simulink model "Ex3sim"  (R2024b)
settings: Solver=VariableStepAuto  StartTime=0.0  StopTime=10.0  RelTol=1e-3
values from neighbouring files (symbols this model uses):
  Ao = phi-L*H    [Ex2.m]    (also in Ex3.m; Extended_Estimator.m = Ae-L*Ce)
  Bo = [gamma L]    [Ex2.m]    (also in Ex3.m; Extended_Estimator.m = [Be L])
  Co = eye(2)    [Ex2.m]    (also in Ex3.m; Extended_Estimator.m = eye(5))
  Do = zeros(2,2)    [Ex2.m]    (also in Ex3.m; Extended_Estimator.m = zeros(5,2))
  k = acker(phi, gamma,eigs_d)    [Ex2.m]    (also in Ex3.m = dlqr(phi_e,gamma_e,Q,R); Ex4.m = acker(A_z,B_z,eigs); Extended_Estimator.m = acker(A,B,pol_c))
  N_u = gains(3)    [Ex2.m]    (also in Ex3.m)
  N_x = gains(1:2)    [Ex2.m]    (also in Ex3.m)
  t_s = 0.001    [Ex2.m]    (also in Ex3.m = 1e-05; Ex4.m = 0.2)
undefined symbols (not defined in the file or in its folder): DiscIntNeverNeededParam
settings Model: Creator=bmm1  LastModifiedBy=bmm1

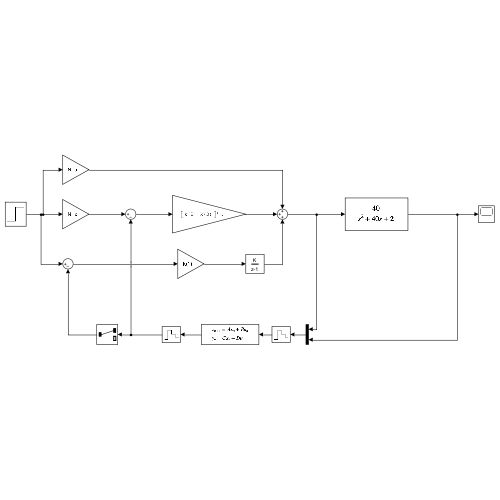
[thumbnail: Simulink's stored preview of the top-level diagram]
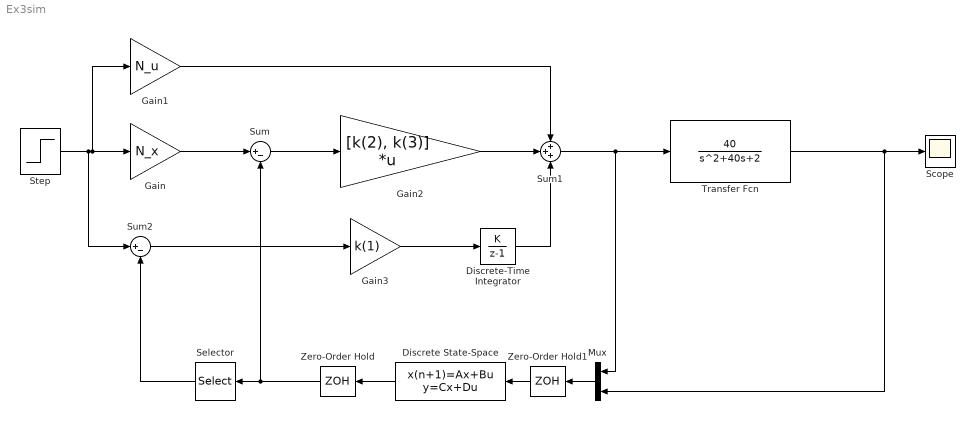
== system Ex3sim ==
  Discrete State-Space : DiscreteStateSpace  A=Ao  B=Bo  C=Co  D=Do  SampleTime=t_s
  Discrete-Time Integrator : DiscreteIntegrator  IntegratorMethod=Accumulation: Forward Euler  SampleTime=t_s  ICPrevOutput=DiscIntNeverNeededParam  ICPrevScaledInput=DiscIntNeverNeededParam
  Gain : Gain  Gain=N_x
  Gain1 : Gain  Gain=N_u
  Gain2 : Gain  Gain=[k(2), k(3)]  Multiplication=Matrix(K*u)
  Gain3 : Gain  Gain=k(1)
  Mux : Mux  Inputs=2
  Scope : Scope
  Selector : Selector  InputPortWidth=2  IndexOptions=Index vector (dialog)  Indices=[1]  OutputSizes=1
  Step : Step  SampleTime=0
  Sum : Sum  Inputs=|+-
  Sum1 : Sum  Inputs=+++
  Sum2 : Sum  Inputs=|+-
  Transfer Fcn : TransferFcn  Numerator=[40]  Denominator=[1 40 2]
  Zero-Order Hold : ZeroOrderHold  SampleTime=t_s
  Zero-Order Hold1 : ZeroOrderHold  SampleTime=t_s
  wires:
  Discrete-Time Integrator/1 -> Sum1/3
  Gain2/1 -> Sum1/2
  Gain1/1 -> Sum1/1
  Sum1/1 -> Mux/1, Transfer Fcn/1
  Transfer Fcn/1 -> Scope/1, Mux/2
  Mux/1 -> Zero-Order Hold1/1
  Step/1 -> Sum2/1, Gain1/1, Gain/1
  Gain/1 -> Sum/1
  Discrete State-Space/1 -> Zero-Order Hold/1
  Sum/1 -> Gain2/1
  Gain3/1 -> Discrete-Time Integrator/1
  Sum2/1 -> Gain3/1
  Selector/1 -> Sum2/2
  Zero-Order Hold/1 -> Sum/2, Selector/1
  Zero-Order Hold1/1 -> Discrete State-Space/1
